simulink model "System_sim"  (R2022b)
settings: Solver=VariableStepAuto  StartTime=0.0  StopTime=10  RelTol=1e-3
PreLoadFcn:
  | param
values from neighbouring files (symbols this model uses):
  b = 0.1    [init_cond.m]    (also in param.m)
  Ce = 1.2    [init_cond.m]    (also in param.m)
  Cm = 1.2    [init_cond.m]    (also in param.m)
  J = 0.04    [init_cond.m]    (also in param.m)
  K_ampl = 10    [param.m]
  K_tach = 0.9    [param.m]
  Lrot = Le+Lf    (= 0.02)    [init_cond.m]    (also in param.m)
  R1 = 680    [init_cond.m]    (also in param.m = 10000)
  R2 = 2*10^3    (= 2000)    [init_cond.m]    (also in param.m)
  R3 = R2    (= 2000)    [init_cond.m]    (also in param.m)
  RF = 20*10^3    (= 20000)    [init_cond.m]    (also in param.m)
  Rrot = Re+Rf    (= 4.9)    [init_cond.m]    (also in param.m)
  TF = RF*CF    (= 0.102)    [init_cond.m]    (also in param.m)
libraries: fl_lib x19, nesl_utility x4, ee_lib x1
settings Model: Creator=antsupove  LastModifiedBy=antsupove
settings DebuggingCC: UnconnectedInputMsg=warning  UnconnectedOutputMsg=warning  UnconnectedLineMsg=warning
settings ModelReferenceCC: EnableRefExpFcnMdlSchedulingChecks=on
settings RTWCC: DLArmComputeVersion=19.05

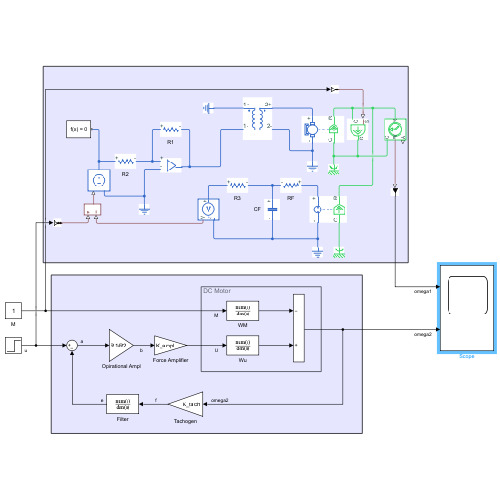
[thumbnail: Simulink's stored preview of the top-level diagram]
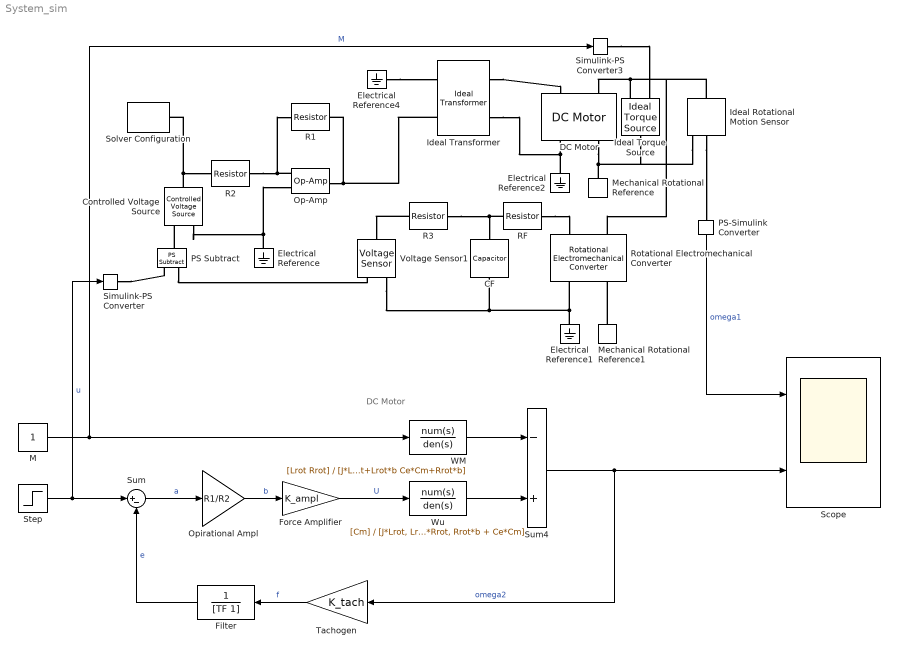
== system System_sim ==
  note: DC Motor
  CF : fl_lib/Electrical/Electrical Elements/Capacitor  c=CF F  r=1e-6 Ohm  g=0 1/Ohm  i_specify=off  i_priority=None  i=0 A  i_nominal_specify=off  i_nominal_unit=A  i_nominal_value=1  v_specify=off  v_priority=None  v=0 V  v_nominal_specify=off  v_nominal_unit=V  v_nominal_value=1  vc_specify=off  vc_priority=High  vc=0 V  vc_nominal_specify=off  vc_nominal_unit=V  vc_nominal_value=1
  Controlled Voltage Source : fl_lib/Electrical/Electrical Sources/Controlled Voltage Source
  DC Motor : ee_lib/Electromechanical/Brushed Motors/DC Motor  field_option=ee.enum.field_option.pm  Rf=100 Ohm  Lf=1 H  Laf=0.15 H  If0=0 A  parameterization=ee.enum.dcparam_option.circuit_param  Ra=Rrot Ohm  La=Lrot H  emf_or_torque=ee.enum.emf_or_torque.ki  Kv=0.072e-3 V/rpm  Ki=Cm N*m/A  T_stall=0.24e-3 N*m  w_max=19100 rpm  w_rated=15000 rpm  P_rated=0.08 W  V_rated=1.5 V  lam_param=ee.enum.lam_param.damping  i_noload=0 A  V_i_noload=1.5 V  J=J kg*m^2  lam=b N*m/(rad/s)  speed0=0 rpm  enable_fault_armature=simscape.enum.onoff.off  rev_faulted=1 / 3  G_faulted_armature=1e-5 S  fault_trigger_armature=ee.enum.faults.faultTrigger.temporal  t_fault_armature=1 s  max_permissible_current_armature=inf A  t_fail_on_current_armature=1 s  enable_fault_field=simscape.enum.onoff.off  G_faulted_field=1e-5 S  fault_trigger_field=ee.enum.faults.faultTrigger.temporal  t_fault_field=1 s  max_permissible_current_field=inf A  t_fail_on_current_field=1 s  fault_action=simscape.enum.assert.action.none  alpha=3.93e-3 1/K  Tmeas=25 degC  thermal_mass=100 J/K  initial_temperature=25 degC
  Electrical Reference{,1..2,4} (4 alike) : fl_lib/Electrical/Electrical Elements/Electrical Reference
  Filter : TransferFcn  Denominator=[TF 1]
  Force Amplifier : Gain  Gain=K_ampl
  Ideal Rotational Motion Sensor : fl_lib/Mechanical/Mechanical Sensors/Ideal Rotational Motion Sensor  reference=foundation.enum.MeasurementReference.difference  acceleration_port=false  velocity_port=true  position_port=true  wrap_angle=simscape.enum.onoff.off  offset=0 rad
  Ideal Torque Source : fl_lib/Mechanical/Mechanical Sources/Ideal Torque Source
  Ideal Transformer : fl_lib/Electrical/Electrical Elements/Ideal Transformer  n=1/K_ampl  i1_specify=off  i1_priority=None  i1=0 A  i1_nominal_specify=off  i1_nominal_unit=A  i1_nominal_value=1  v1_specify=off  v1_priority=None  v1=0 V  v1_nominal_specify=off  v1_nominal_unit=V  v1_nominal_value=1  i2_specify=off  i2_priority=None  i2=0 A  i2_nominal_specify=off  i2_nominal_unit=A  i2_nominal_value=1  v2_specify=off  v2_priority=None  v2=0 V  v2_nominal_specify=off  v2_nominal_unit=V  v2_nominal_value=1
  M : Constant
  Mechanical Rotational Reference : fl_lib/Mechanical/Rotational Elements/Mechanical Rotational Reference
  Mechanical Rotational Reference1 : fl_lib/Mechanical/Rotational Elements/Mechanical Rotational Reference
  Op-Amp : fl_lib/Electrical/Electrical Elements/Op-Amp  outI_specify=off  outI_priority=None  outI=0 A  outI_nominal_specify=off  outI_nominal_unit=A  outI_nominal_value=1
  Opirational Ampl : Gain  Gain=R1/R2
  PS Subtract : fl_lib/Physical Signals/Functions/PS Subtract
  PS-Simulink Converter : nesl_utility/PS-Simulink Converter  PhysicalDomain=network_engine_domain  SubClassName=ps_output  LeftPortType=input  RightPortType=output  PseudoPeriodic=off  Frequencies=[]  VectorFormat=1-D array  Unit=inherit  AffineConversion=off
  R1 : fl_lib/Electrical/Electrical Elements/Resistor  R=R1 Ohm  i_specify=off  i_priority=None  i=0 A  i_nominal_specify=off  i_nominal_unit=A  i_nominal_value=1  v_specify=off  v_priority=None  v=0 V  v_nominal_specify=off  v_nominal_unit=V  v_nominal_value=1
  R2 : fl_lib/Electrical/Electrical Elements/Resistor  R=R2 Ohm  i_specify=off  i_priority=None  i=0 A  i_nominal_specify=off  i_nominal_unit=A  i_nominal_value=1  v_specify=off  v_priority=None  v=0 V  v_nominal_specify=off  v_nominal_unit=V  v_nominal_value=1
  R3 : fl_lib/Electrical/Electrical Elements/Resistor  R=R3 Ohm  i_specify=off  i_priority=None  i=0 A  i_nominal_specify=off  i_nominal_unit=A  i_nominal_value=1  v_specify=off  v_priority=None  v=0 V  v_nominal_specify=off  v_nominal_unit=V  v_nominal_value=1
  RF : fl_lib/Electrical/Electrical Elements/Resistor  R=RF Ohm  i_specify=off  i_priority=None  i=0 A  i_nominal_specify=off  i_nominal_unit=A  i_nominal_value=1  v_specify=off  v_priority=None  v=0 V  v_nominal_specify=off  v_nominal_unit=V  v_nominal_value=1
  Rotational Electromechanical Converter : fl_lib/Electrical/Electrical Elements/Rotational Electromechanical Converter  K=K_tach V/(rad/s)  i_specify=off  i_priority=None  i=0 A  i_nominal_specify=off  i_nominal_unit=A  i_nominal_value=1  v_specify=off  v_priority=None  v=0 V  v_nominal_specify=off  v_nominal_unit=V  v_nominal_value=1  t_specify=off  t_priority=None  t=0 N*m  t_nominal_specify=off  t_nominal_unit=N*m  t_nominal_value=1  w_specify=off  w_priority=None  w=0 rad/s  w_nominal_specify=off  w_nominal_unit=rad/s  w_nominal_value=1
  Scope : Scope  NumInputPorts=2
  Simulink-PS Converter : nesl_utility/Simulink-PS Converter  PhysicalDomain=network_engine_domain  SubClassName=ps_input  LeftPortType=input  RightPortType=output  PseudoPeriodic=off  Frequencies=[]  NoiseDistribution=none  NoiseParameters=[]  Unit=V  AffineConversion=off  FilteringAndDerivatives=filter  SimscapeFilterOrder=2  InputFilterTimeConstant=0.001  UdotUserProvided=0
  Simulink-PS Converter3 : nesl_utility/Simulink-PS Converter  PhysicalDomain=network_engine_domain  SubClassName=ps_input  LeftPortType=input  RightPortType=output  PseudoPeriodic=off  Frequencies=[]  NoiseDistribution=none  NoiseParameters=[]  Unit=1  AffineConversion=off  FilteringAndDerivatives=filter  SimscapeFilterOrder=2  InputFilterTimeConstant=0.001  UdotUserProvided=0
  Solver Configuration : nesl_utility/Solver Configuration  PhysicalDomain=network_engine_domain  SubClassName=solver  LeftPortType=input  RightPortType=generic  Tones=[]  Harmonics=[]  SimulateNoise=off  Profile=off  UseLocalSampling=off  EnableSwitchedLinearOptims=on  FrequencyDomain=off  UseCCode=off  RelTol=0.001  AbsTol=1e-06  MinStep=1e-09  ToWorkspace=off  RevertToSquareIcSolve=off  NumHomotopyIterations=100  PhasorMode=off  PhasorModeNumHarmonics=1  ConsistencySolver=NEWTON_FTOL  IndexReductionMethod=DerivativeReplacement  DoDC=off  ResidualTolerance=1e-09  ConsistencyTolSource=GLOBAL  ConsistencyAbsTol=0.001  ConsistencyRelTol=0.001  ConsistencyTolFactor=0.001  UseLocalSolver=off  LocalSolverChoice=NE_BACKWARD_EULER_ADVANCER  ResolveIndetEquations=on  FunctionEvalNumThread=1  LocalSolverSampleTime=0.001  DoFixedCost=off  MaxNonlinIter=3  MaxModeIter=2  ComputeImpulses=off  ImpulseIterations=2  LinearAlgebra=auto  LinearAlgebraNumThread=0  EquationFormulation=NE_TIME_EF  DelaysMemoryBudget=1024  AutomaticFiltering=on  FilteringTimeConstant=0.001  PartitionStorageMethod=AS_NEEDED  PartitionMemoryBudget=1024  PartitionMethod=ROBUST
  Step : Step  SampleTime=0
  Sum : Sum  Inputs=|+-
  Sum4 : Sum  Inputs=-+
  Tachogen : Gain  Gain=K_tach
  Voltage Sensor1 : fl_lib/Electrical/Electrical Sensors/Voltage Sensor
  WM : TransferFcn  Numerator=[Lrot Rrot]  Denominator=[J*Lrot J*Rrot+Lrot*b Ce*Cm+Rrot*b]
  Wu : TransferFcn  Numerator=[Cm]  Denominator=[J*Lrot, Lrot*b + J*Rrot, Rrot*b + Ce*Cm]
  wires:
  WM/1 -> Sum4/1
  Wu/1 -> Sum4/2
  Tachogen/1 -> Filter/1  "f"
  Step/1 -> Simulink-PS Converter/1, Sum/1  "u"
  Sum/1 -> Opirational Ampl/1  "a"
  Opirational Ampl/1 -> Force Amplifier/1  "b"
  Force Amplifier/1 -> Wu/1  "U"
  M/1 -> WM/1, Simulink-PS Converter3/1  "M"
  Sum4/1 -> Tachogen/1, Scope/2  "omega2"
  Filter/1 -> Sum/2  "e"
  PS-Simulink Converter/1 -> Scope/1  "omega1"
  connections:
  Electrical Reference/LConn1 -- Controlled Voltage Source/RConn2 -- Op-Amp/LConn2
  R2/RConn1 -- Op-Amp/LConn1 -- R1/LConn1
  Op-Amp/RConn1 -- Ideal Transformer/LConn2 -- R1/RConn1
  Simulink-PS Converter/RConn1 -- PS Subtract/LConn1
  Electrical Reference1/LConn1 -- Voltage Sensor1/RConn2 -- CF/RConn1 -- Rotational Electromechanical Converter/RConn1
  RF/LConn1 -- Rotational Electromechanical Converter/LConn1
  Controlled Voltage Source/LConn1 -- Solver Configuration/RConn1 -- R2/LConn1
  Electrical Reference2/LConn1 -- Ideal Transformer/RConn2 -- DC Motor/RConn1
  Mechanical Rotational Reference/LConn1 -- DC Motor/RConn2 -- Ideal Rotational Motion Sensor/RConn1 -- Ideal Torque Source/LConn1
  Ideal Torque Source/RConn2 -- Ideal Rotational Motion Sensor/LConn1 -- Rotational Electromechanical Converter/LConn2 -- DC Motor/LConn2
  Ideal Rotational Motion Sensor/RConn2 -- PS-Simulink Converter/LConn1
  Simulink-PS Converter3/RConn1 -- Ideal Torque Source/RConn1
  RF/RConn1 -- R3/RConn1 -- CF/LConn1
  Mechanical Rotational Reference1/LConn1 -- Rotational Electromechanical Converter/RConn2
  Ideal Transformer/RConn1 -- DC Motor/LConn1
  Electrical Reference4/LConn1 -- Ideal Transformer/LConn1
  PS Subtract/RConn1 -- Controlled Voltage Source/RConn1
  PS Subtract/LConn2 -- Voltage Sensor1/RConn1
  R3/LConn1 -- Voltage Sensor1/LConn1
